simulink model "sim_regulatory"  (R2022b)
settings: Solver=VariableStepAuto  StartTime=0.0  StopTime=1000.0  RelTol=1e-3
values from neighbouring files (symbols this model uses):
  Kc = 1/K*(tau/td)*(0.9 + td/(12*tau))    [assign7.m]
  taui = (td*(30 + (3*td)/tau))/(9 + (20*td)/tau)    [assign7.m]
settings Model: Creator=Administrator  LastModifiedBy=Administrator

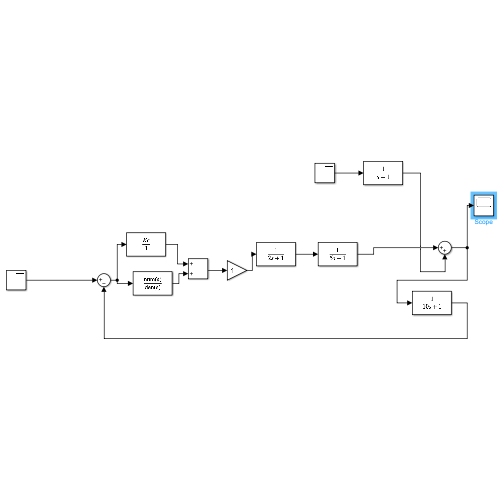
[thumbnail: Simulink's stored preview of the top-level diagram]
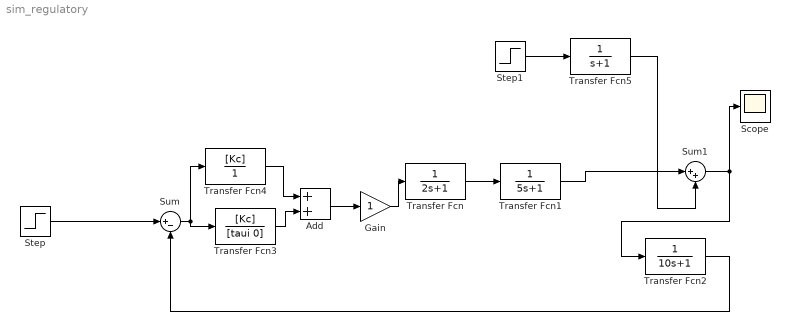
== system sim_regulatory ==
  Add : Sum
  Gain : Gain
  Scope : Scope
  Step : Step  Time=0  After=0  SampleTime=0
  Step1 : Step  SampleTime=0
  Sum : Sum  Inputs=|+-
  Sum1 : Sum  Inputs=|++
  Transfer Fcn : TransferFcn  Denominator=[2 1]
  Transfer Fcn1 : TransferFcn  Denominator=[5 1]
  Transfer Fcn2 : TransferFcn  Denominator=[10 1]
  Transfer Fcn3 : TransferFcn  Numerator=[Kc]  Denominator=[taui 0]
  Transfer Fcn4 : TransferFcn  Numerator=[Kc]  Denominator=[0 1]
  Transfer Fcn5 : TransferFcn  Denominator=[1 1]
  wires:
  Add/1 -> Gain/1
  Sum/1 -> Transfer Fcn4/1, Transfer Fcn3/1
  Transfer Fcn3/1 -> Add/2
  Transfer Fcn4/1 -> Add/1
  Gain/1 -> Transfer Fcn/1
  Step/1 -> Sum/1
  Transfer Fcn2/1 -> Sum/2
  Transfer Fcn/1 -> Transfer Fcn1/1
  Transfer Fcn1/1 -> Sum1/1
  Step1/1 -> Transfer Fcn5/1
  Transfer Fcn5/1 -> Sum1/2
  Sum1/1 -> Transfer Fcn2/1, Scope/1
